simulink model "InteractiveArmModel_R2021a_v1"  (R2021a)
settings: Solver=ode4  StartTime=0.0  StopTime=3000  FixedStep=1/150  MaxStep=1/50  MinStep=1/200  RelTol=1e-5  AbsTol=1e-6  EnableMultiTasking=on
model workspace (MAT data in the model file):
  MaxEccentricFlexor = 0.5
  PoleZ = 0.85
  SampleTime = 0.05
  musNoise = 0
  musNoiseLevel : Simulink.Parameter (value not decoded)
libraries: simulink x1
(part 2 of 3)

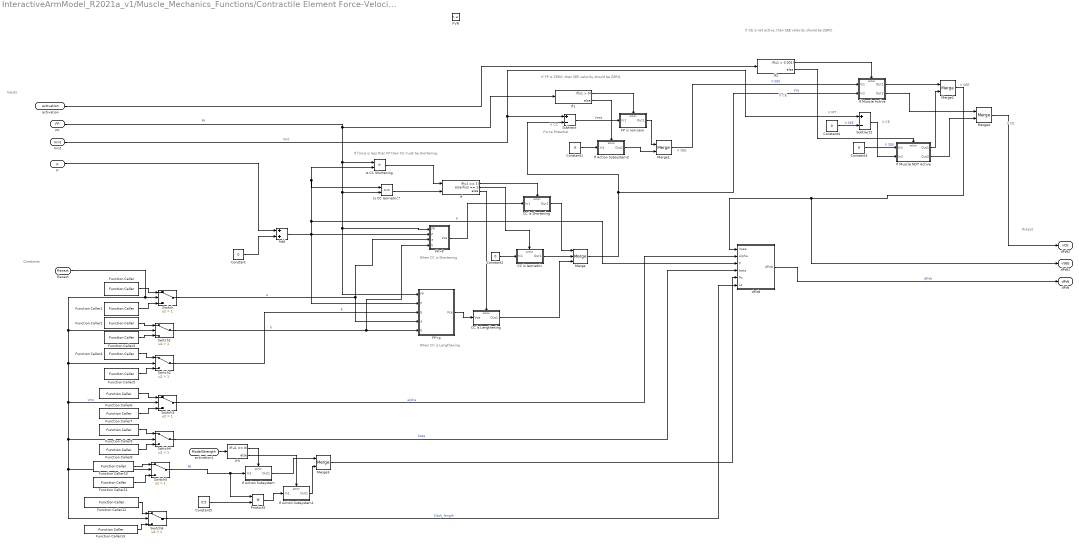
== system InteractiveArmModel_R2021a_v1/Muscle_Mechanics_Functions/Contractile Element Force-Velocity Relation ==
  note: V CE
  note: V MT
  note: V SEE
  note: V CE
  note: V CE
  note: V CC
  note: V SEE
  note: If force is less than FP then CC must be shortening.
  note: When CC is Shortening
  note: When CC is Lengthening
  note: Force Potential
  note: Output
  note: Inputs
  note: Constants
  note: If FP is ZERO, then SEE velocity should be ZERO.
  note: If CE is not active, then SEE velocity should be ZERO.
  FVR : TriggerPort  TriggerType=function-call  IsSimulinkFunction=on  FunctionName=FVR  FunctionVisibility=scoped  VariantControl=(inherit)
  Add : Sum
  CC is Isometric : Subsystem  TreatAsAtomicUnit=on
  CC is Lengthening : Subsystem  TreatAsAtomicUnit=on
  CC is Shortening : Subsystem  TreatAsAtomicUnit=on
  Constant{,1..4} (5 alike) : Constant  Value=0
  Constant5 : Constant  Value=0.5
  FP is non-zero : Subsystem  TreatAsAtomicUnit=on
  FP<p : Subsystem
  FP>P : Subsystem
  Function Caller : FunctionCaller  FunctionPrototype=y = Constants.aF()  InputArgumentSpecifications=<Enter example>  OutputArgumentSpecifications=<Enter example>
  Function Caller1 : FunctionCaller  FunctionPrototype=y = Constants.aE()  InputArgumentSpecifications=<Enter example>  OutputArgumentSpecifications=<Enter example>
  Function Caller10 : FunctionCaller  FunctionPrototype=y = Constants.P0F()  InputArgumentSpecifications=<Enter example>  OutputArgumentSpecifications=<Enter example>
  Function Caller11 : FunctionCaller  FunctionPrototype=y = Constants.P0E()  InputArgumentSpecifications=<Enter example>  OutputArgumentSpecifications=<Enter example>
  Function Caller12 : FunctionCaller  FunctionPrototype=y = Constants.Slack_lengthF()  InputArgumentSpecifications=<Enter example>  OutputArgumentSpecifications=<Enter example>
  Function Caller13 : FunctionCaller  FunctionPrototype=y = Constants.Slack_lengthE()  InputArgumentSpecifications=<Enter example>  OutputArgumentSpecifications=<Enter example>
  Function Caller2 : FunctionCaller  FunctionPrototype=y = Constants.bF()  InputArgumentSpecifications=<Enter example>  OutputArgumentSpecifications=<Enter example>
  Function Caller3 : FunctionCaller  FunctionPrototype=y = Constants.bE()  InputArgumentSpecifications=<Enter example>  OutputArgumentSpecifications=<Enter example>
  Function Caller4 : FunctionCaller  FunctionPrototype=y = Constants.EF()  InputArgumentSpecifications=<Enter example>  OutputArgumentSpecifications=<Enter example>
  Function Caller5 : FunctionCaller  FunctionPrototype=y = Constants.EE()  InputArgumentSpecifications=<Enter example>  OutputArgumentSpecifications=<Enter example>
  Function Caller6 : FunctionCaller  FunctionPrototype=y = Constants.alphaF()  InputArgumentSpecifications=<Enter example>  OutputArgumentSpecifications=<Enter example>
  Function Caller7 : FunctionCaller  FunctionPrototype=y = Constants.alphaE()  InputArgumentSpecifications=<Enter example>  OutputArgumentSpecifications=<Enter example>
  Function Caller8 : FunctionCaller  FunctionPrototype=y = Constants.betaE()  InputArgumentSpecifications=<Enter example>  OutputArgumentSpecifications=<Enter example>
  Function Caller9 : FunctionCaller  FunctionPrototype=y = Constants.betaF()  InputArgumentSpecifications=<Enter example>  OutputArgumentSpecifications=<Enter example>
  If : If  NumInputs=2  IfExpression=u1 == 1  ElseIfExpressions=u2 == 1
  If Action Subsystem : Subsystem  TreatAsAtomicUnit=on
  If Action Subsystem1 : Subsystem  TreatAsAtomicUnit=on
  If Action Subsystem3 : Subsystem  TreatAsAtomicUnit=on
  If Muscle Active : Subsystem  TreatAsAtomicUnit=on
  If Muscle NOT Active : Subsystem  TreatAsAtomicUnit=on
  If1 : If
  If2 : If  IfExpression=u1 > 0.001
  If3 : If  IfExpression=u1 == 0
  Is CC Isometric? : RelationalOperator  Operator===  OutDataTypeStr=boolean  RndMeth=Simplest
  Is CC Shortening : RelationalOperator  Operator=>  OutDataTypeStr=boolean  RndMeth=Simplest
  Merge : Merge  Inputs=3
  Merge{1..4} (4 alike) : Merge
  Product5 : Product
  Subtract : Sum  Inputs=+-
  Subtract2 : Sum  Inputs=+-
  Switch{,1..6} (7 alike) : Switch  Criteria=u2 > Threshold  Threshold=1
  dP/dt : Subsystem
  FP : ArgIn  DisableCoverage=on  ArgumentName=FP
  Vmt : ArgIn  DisableCoverage=on  Port=2  ArgumentName=Vmt
  p : ArgIn  DisableCoverage=on  Port=3  ArgumentName=p
  flexext : ArgIn  DisableCoverage=on  Port=4  ArgumentName=flexext
  activation : ArgIn  DisableCoverage=on  Port=5  ArgumentName=activation
  activation1 : ArgIn  DisableCoverage=on  Port=6  ArgumentName=ModelStrength
  dPdt1 : ArgOut  DisableCoverage=on  ArgumentName=vSEE
  dPdt : ArgOut  DisableCoverage=on  Port=2  ArgumentName=dPdt
  dPdt2 : ArgOut  DisableCoverage=on  Port=3  ArgumentName=vCE
  wires:
  FP/1 -> If1/1, Is CC Shortening/1, Is CC Isometric?/2, FP<p/1(FP), FP>P/1(FP)  "FP"
  Switch2/1 -> FP<p/3(E)  "E"
  Switch1/1 -> FP>P/4(b), FP<p/5(b)  "b"
  FP<p/1(Vce) -> CC is Lengthening/1(Vce)
  FP>P/1(Vce) -> CC is Shortening/1(In1)
  Merge/1 -> If Muscle Active/2(In2), Subtract/2  "Vce"
  Switch/1 -> FP>P/3(a), FP<p/4(a)  "a"
  If/1 -> CC is Shortening/Action
  dP/dt/1(dP/dt) -> dPdt/1  "dP/dt"
  Switch4/1 -> dP/dt/4(beta)  "beta"
  If/3 -> CC is Lengthening/Action
  Is CC Shortening/1 -> If/1
  Switch3/1 -> dP/dt/2(alpha)  "alpha"
  Constant/1 -> Add/2
  CC is Shortening/1(Out1) -> Merge/1
  Switch6/1 -> dP/dt/6(Ls)  "Slack_length"
  Vmt/1 -> Subtract2/1, Subtract/1  "Vmt"
  CC is Lengthening/1(Out1) -> Merge/3
  Is CC Isometric?/1 -> If/2
  If/2 -> CC is Isometric/Action
  Constant2/1 -> CC is Isometric/1(In1)
  p/1 -> Add/1
  Function Caller1/1 -> Switch/3
  Function Caller/1 -> Switch/1
  flexext/1 -> Switch/2, Switch5/2, Switch6/2, Switch4/2, Switch3/2, Switch2/2, Switch1/2  "Vmt"
  Function Caller2/1 -> Switch1/1
  Function Caller3/1 -> Switch1/3
  Function Caller4/1 -> Switch2/1
  Function Caller5/1 -> Switch2/3
  Function Caller6/1 -> Switch3/1
  Function Caller7/1 -> Switch3/3
  Function Caller9/1 -> Switch4/1
  Function Caller8/1 -> Switch4/3
  Function Caller10/1 -> Switch5/1
  Function Caller11/1 -> Switch5/3
  Function Caller13/1 -> Switch6/3
  Function Caller12/1 -> Switch6/1
  Subtract/1 -> FP is non-zero/1(In1)  "Vsee"
  If1/1 -> FP is non-zero/Action
  If1/2 -> If Action Subsystem3/Action
  Constant1/1 -> If Action Subsystem3/1(In1)
  FP is non-zero/1(Out1) -> Merge1/1
  If Action Subsystem3/1(Out1) -> Merge1/2
  activation/1 -> If2/1
  If2/1 -> If Muscle Active/Action
  If2/2 -> If Muscle NOT Active/Action
  Merge1/1 -> If Muscle Active/1(In1)  "V SEE"
  Constant3/1 -> If Muscle NOT Active/1(In1)  "V SEE"
  If Muscle Active/1(Out1) -> Merge2/1
  If Muscle NOT Active/1(Out1) -> Merge2/2
  Merge2/1 -> dPdt1/1, dP/dt/1(Vsee)
  CC is Isometric/1(Out1) -> Merge/2
  Add/1 -> Is CC Shortening/2, Is CC Isometric?/1, dP/dt/3(P), FP<p/2(P), FP>P/2(P)  "P"
  Subtract2/1 -> If Muscle NOT Active/2(In2)
  If Muscle Active/2(Out2) -> Merge4/1
  If Muscle NOT Active/2(Out2) -> Merge4/2
  Merge4/1 -> dPdt2/1
  Constant4/1 -> Subtract2/2  "V SEE"
  Merge3/1 -> dP/dt/5(Po)
  Switch5/1 -> Product5/1, If Action Subsystem/1(In1)  "P0"
  activation1/1 -> If3/1
  If3/1 -> If Action Subsystem/Action
  If Action Subsystem/1(Out1) -> Merge3/1
  Constant5/1 -> Product5/2
  Product5/1 -> If Action Subsystem1/1(In1)
  If3/2 -> If Action Subsystem1/Action
  If Action Subsystem1/1(Out1) -> Merge3/2

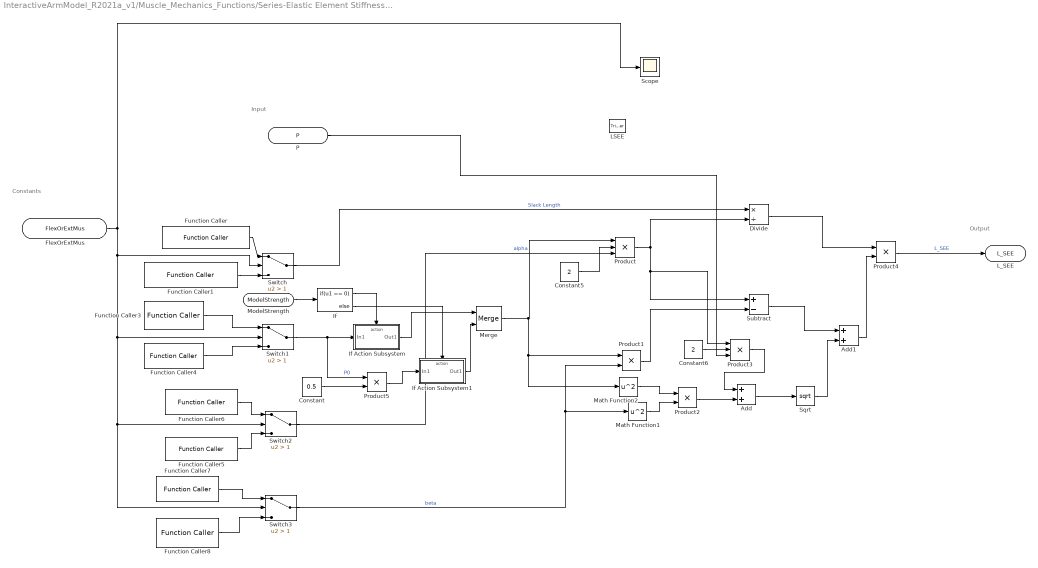
== system InteractiveArmModel_R2021a_v1/Muscle_Mechanics_Functions/Series-Elastic Element Stiffness Relation  ==
  note: Output
  note: Input
  note: Constants
  LSEE : TriggerPort  TriggerType=function-call  IsSimulinkFunction=on  FunctionName=LSEE  FunctionVisibility=scoped  VariantControl=(inherit)
  Add : Sum
  Add1 : Sum
  Constant : Constant  Value=0.5
  Constant5 : Constant  Value=2
  Constant6 : Constant  Value=2
  Divide : Product  Inputs=*/
  Function Caller : FunctionCaller  FunctionPrototype=y = Constants.Slack_lengthF()  InputArgumentSpecifications=<Enter example>  OutputArgumentSpecifications=<Enter example>
  Function Caller1 : FunctionCaller  FunctionPrototype=y = Constants.Slack_lengthE()  InputArgumentSpecifications=<Enter example>  OutputArgumentSpecifications=<Enter example>
  Function Caller3 : FunctionCaller  FunctionPrototype=y = Constants.P0F()  InputArgumentSpecifications=<Enter example>  OutputArgumentSpecifications=<Enter example>
  Function Caller4 : FunctionCaller  FunctionPrototype=y = Constants.P0E()  InputArgumentSpecifications=<Enter example>  OutputArgumentSpecifications=<Enter example>
  Function Caller5 : FunctionCaller  FunctionPrototype=y = Constants.alphaE()  InputArgumentSpecifications=<Enter example>  OutputArgumentSpecifications=<Enter example>
  Function Caller6 : FunctionCaller  FunctionPrototype=y = Constants.alphaF()  InputArgumentSpecifications=<Enter example>  OutputArgumentSpecifications=<Enter example>
  Function Caller7 : FunctionCaller  FunctionPrototype=y = Constants.betaF()  InputArgumentSpecifications=<Enter example>  OutputArgumentSpecifications=<Enter example>
  Function Caller8 : FunctionCaller  FunctionPrototype=y = Constants.betaE()  InputArgumentSpecifications=<Enter example>  OutputArgumentSpecifications=<Enter example>
  If : If  IfExpression=u1 == 0
  If Action Subsystem : Subsystem  TreatAsAtomicUnit=on
  If Action Subsystem1 : Subsystem  TreatAsAtomicUnit=on
  Math Function1 : Math  Operator=square  SaturateOnIntegerOverflow=on
  Math Function2 : Math  Operator=square  SaturateOnIntegerOverflow=on
  Merge : Merge
  Product : Product  Inputs=3
  Product{1..2,4..5} (4 alike) : Product
  Product3 : Product  Inputs=3
  Scope : Scope
  Sqrt : Sqrt  SaturateOnIntegerOverflow=on
  Subtract : Sum  Inputs=+-
  Switch{,1..3} (4 alike) : Switch  Criteria=u2 > Threshold  Threshold=1
  P : ArgIn  DisableCoverage=on  ArgumentName=P
  FlexOrExtMus : ArgIn  DisableCoverage=on  Port=2  ArgumentName=FlexOrExtMus
  ModelStrength : ArgIn  DisableCoverage=on  Port=3  ArgumentName=ModelStrength
  L_SEE : ArgOut  DisableCoverage=on  ArgumentName=L_SEE
  wires:
  P/1 -> Product3/3
  Product3/1 -> Add/1
  Product2/1 -> Add/2
  Math Function2/1 -> Product2/1
  Constant5/1 -> Product/2
  Product4/1 -> L_SEE/1  "L_SEE"
  Constant6/1 -> Product3/2
  Product/1 -> Divide/2, Product3/1, Subtract/1
  Sqrt/1 -> Add1/2
  Add1/1 -> Product4/2
  Switch3/1 -> Math Function1/1, Product1/2  "beta"
  Subtract/1 -> Add1/1
  Switch2/1 -> Product/3  "alpha"
  Math Function1/1 -> Product2/2
  Add/1 -> Sqrt/1
  Switch/1 -> Divide/1  "Slack Length"
  Divide/1 -> Product4/1
  Product1/1 -> Subtract/2
  Function Caller/1 -> Switch/1
  Function Caller1/1 -> Switch/3
  Function Caller3/1 -> Switch1/1
  Function Caller4/1 -> Switch1/3
  Function Caller6/1 -> Switch2/1
  Function Caller5/1 -> Switch2/3
  Function Caller8/1 -> Switch3/3
  Function Caller7/1 -> Switch3/1
  FlexOrExtMus/1 -> Switch3/2, Switch2/2, Switch1/2, Switch/2, Scope/1
  ModelStrength/1 -> If/1
  Switch1/1 -> Product5/1, If Action Subsystem/1(In1)  "P0"
  If/1 -> If Action Subsystem/Action
  If/2 -> If Action Subsystem1/Action
  Constant/1 -> Product5/2
  Product5/1 -> If Action Subsystem1/1(In1)
  If Action Subsystem/1(Out1) -> Merge/1
  If Action Subsystem1/1(Out1) -> Merge/2
  Merge/1 -> Math Function2/1, Product1/1, Product/1

== system InteractiveArmModel_R2021a_v1/Trial Start//Stop//Increment Control/Counter for Trial Number ==
  Trigger : TriggerPort  VariantControl=Variant
  Add : Sum
  Constant : Constant  Value=0
  Delay : Delay  DelayLength=1  InitialCondition=0
  Increment Stored Integer : simulink/Additional Math & Discrete/Additional Math: Increment - Decrement/Increment Stored Integer
  Trial Number Switch : Outport
  wires:
  Constant/1 -> Add/1
  Add/1 -> Increment Stored Integer/1
  Increment Stored Integer/1 -> Trial Number Switch/1, Delay/1
  Delay/1 -> Add/2

== system InteractiveArmModel_R2021a_v1/Trial Start//Stop//Increment Control/Extract Movement Time ==
  Trial Time : Inport
  Loop Running Flag : TriggerPort  TriggerType=falling  VariantControl=Variant
  Movement Time : Outport
  wires:
  Trial Time/1 -> Movement Time/1

== system InteractiveArmModel_R2021a_v1/Trial Start//Stop//Increment Control/Flag for What Phase Trial is In ==
  note: Flags
      | Specifying
      | What
      | Phase of Trial
      | Is Model
      | Currentely In
  Trial Time Flag : Inport
  Stop Criteria Flag : Inport  Port=2
  If Action Subsystem5 : Subsystem  TreatAsAtomicUnit=on
  If Action Subsystem6 : Subsystem  TreatAsAtomicUnit=on
  If Action Subsystem7 : Subsystem  TreatAsAtomicUnit=on
  If3 : If  NumInputs=2  IfExpression=u1 == 0  ElseIfExpressions=u2 == 0
  Merge2 : Merge  Inputs=3
  StopCriteriaFlag : Constant  Value=2
  TrialIsRunning : Constant  Value=0
  TrialTimeFlag : Constant
  message display : Outport
  wires:
  If Action Subsystem6/1(Out1) -> Merge2/2
  If Action Subsystem7/1(Out1) -> Merge2/3
  If Action Subsystem5/1(Out1) -> Merge2/1
  TrialTimeFlag/1 -> If Action Subsystem5/1(In1)  "Time is up"
  TrialIsRunning/1 -> If Action Subsystem7/1(In1)  "Keeps running"
  Stop Criteria Flag/1 -> If3/2
  If3/2 -> If Action Subsystem6/Action
  If3/1 -> If Action Subsystem5/Action
  StopCriteriaFlag/1 -> If Action Subsystem6/1(In1)  "Success"
  If3/3 -> If Action Subsystem7/Action
  Trial Time Flag/1 -> If3/1
  Merge2/1 -> message display/1  "message display"

== system InteractiveArmModel_R2021a_v1/Trial Start//Stop//Increment Control/Reset Trigger Logic ==
  note: Reset Trigger
  Trial Time : Inport
  Stop Criteria Flag : Inport  Port=2
  Constant1 : Constant  Value=0
  Logical Operator1 : Logic  AllPortsSameDT=off  OutDataTypeStr=boolean
  Relational Operator : RelationalOperator  Operator=>  OutDataTypeStr=boolean  RndMeth=Simplest
  Reset Trigger : Outport
  wires:
  Relational Operator/1 -> Logical Operator1/1
  Trial Time/1 -> Relational Operator/1
  Constant1/1 -> Relational Operator/2
  Stop Criteria Flag/1 -> Logical Operator1/2
  Logical Operator1/1 -> Reset Trigger/1  "Reset Trigger"

== system InteractiveArmModel_R2021a_v1/Trial Start//Stop//Increment Control/Stop Criteria Flag Control (Between Trials) ==
  note: Immediately goes to zero when stop on target. Switches to 1 at the start of the one-second "get ready" pre-trial wait time.
  note: 0 = Stop criteria Satisfied.
  note: Detect 0 at Stop Criteria, wait for a second, and make that 1 again. If the trial (while loop)
      |  is stopped because of the StopCriteria, this logic makes it start again for the next trial
  Stop Criteria Flag In : Inport
  Constant : Constant
  Data Type Conversion1 : DataTypeConversion
  Delay1 : Delay  DelayLength=100  InitialCondition=0
  Delay2 : Delay  DelayLength=1  InitialCondition=0
  If Action Subsystem3 : Subsystem  TreatAsAtomicUnit=on
  If Action Subsystem4 : Subsystem  TreatAsAtomicUnit=on
  If2 : If  IfExpression=u1 == 0
  Merge1 : Merge
  Stop Criteria Flag Out : Outport
  wires:
  Stop Criteria Flag In/1 -> Delay2/1, Delay1/1
  If Action Subsystem3/1(Out1) -> Merge1/1
  If Action Subsystem4/1(Out1) -> Merge1/2
  If2/1 -> If Action Subsystem3/Action
  Delay1/1 -> If2/1
  Merge1/1 -> Stop Criteria Flag Out/1  "StopCriteria"
  Data Type Conversion1/1 -> If Action Subsystem4/1(In1)
  Delay2/1 -> Data Type Conversion1/1
  If2/2 -> If Action Subsystem4/Action
  Constant/1 -> If Action Subsystem3/1(In1)

== system InteractiveArmModel_R2021a_v1/Trial Start//Stop//Increment Control/Subsystem ==
  note: If 0, then trial time is up or stop criteria is satisfied, so reset the trial time to 0.
  note: Reset the trial time for each trial.
  In1 : Inport
  Digital Clock : DigitalClock  SampleTime=-1
  If : If  IfExpression=u1 == 0  ShowElse=off
  If Action Subsystem : Subsystem  TreatAsAtomicUnit=on
  Subtract : Sum  Inputs=+-
  To Workspace1 : ToWorkspace  VariableName=simulationTime  SampleTime=-1
  To Workspace2 : ToWorkspace  VariableName=trialTime  SampleTime=-1
  Simulation Time : Outport
  Trial Time : Outport  Port=2
  wires:
  Digital Clock/1 -> Simulation Time/1, Subtract/1, If Action Subsystem/1(In1), To Workspace1/1
  If Action Subsystem/1(Out1) -> Subtract/2
  Subtract/1 -> Trial Time/1, To Workspace2/1  "Trial time"
  If/1 -> If Action Subsystem/Action
  In1/1 -> If/1

== system InteractiveArmModel_R2021a_v1/Trial Start//Stop//Increment Control/Subsystem1 ==
  note: Changes to zero if trial time exceeded.
  note: StopCriteria&TrialTime
  Trial Time : Inport
  Stop Criteria Flag : Inport  Port=2
  Logical Operator : Logic  AllPortsSameDT=off  OutDataTypeStr=boolean
  Product : Product
  Relational Operator2 : RelationalOperator  Operator=<  RndMeth=Simplest
  Trial time : Constant  Value=5
  Trial time1 : Constant
  StopCriteria&TrialTime Flag : Outport
  Trial Time Flag : Outport  Port=2
  wires:
  Trial time1/1 -> Product/1
  Relational Operator2/1 -> Product/2
  Stop Criteria Flag/1 -> Logical Operator/2
  Logical Operator/1 -> StopCriteria&TrialTime Flag/1  "StopCriteria&TrialTime"
  Trial time/1 -> Relational Operator2/2
  Product/1 -> Trial Time Flag/1, Logical Operator/1  "Time"
  Trial Time/1 -> Relational Operator2/1

== system InteractiveArmModel_R2021a_v1/Trial Start//Stop//Increment Control/Subsystem2 ==
  note: Make IC 1 for the first 0.01 sec. This is to start the trials.
  Simulation Time : Inport
  StopCriteria&TrialTime Flag : Inport  Port=2
  Constant2 : Constant
  If Action Subsystem1 : Subsystem  TreatAsAtomicUnit=on
  If Action Subsystem2 : Subsystem  TreatAsAtomicUnit=on
  If1 : If  IfExpression=u1 < 0.01
  Merge : Merge
  Product1 : Product
  Trial time2 : Constant
  IC : Outport
  wires:
  If1/1 -> If Action Subsystem1/Action
  Constant2/1 -> If Action Subsystem1/1(In1)
  StopCriteria&TrialTime Flag/1 -> Product1/1
  If Action Subsystem1/1(Out1) -> Merge/1
  If Action Subsystem2/1(Out1) -> Merge/2
  Trial time2/1 -> Product1/2
  Merge/1 -> IC/1  "IC"
  Product1/1 -> If Action Subsystem2/1(In1)  "Time"
  If1/2 -> If Action Subsystem2/Action
  Simulation Time/1 -> If1/1

== system InteractiveArmModel_R2021a_v1/While Loop (Main Simulation Code)/Actuator Selection Logic ==
  Control Input : Inport
  Add2 : Sum
  Constant{,1..3,5..6} (6 alike) : Constant  Value=0
  Constant4 : Constant
  Function Caller : FunctionCaller  FunctionPrototype=y = Constants.ActuatorType()  InputArgumentSpecifications=<Enter example>  OutputArgumentSpecifications=<Enter example>
  Multiport Switch : MultiPortSwitch
  Multiport Switch1 : MultiPortSwitch
  Multiport Switch2 : MultiPortSwitch
  Torque Control Signal : Outport
  Force Actuator Control Signal : Outport  Port=2
  MuscleControlSignal : Outport  Port=3
  wires:
  Add2/1 -> Multiport Switch/1, Multiport Switch2/1, Multiport Switch1/1
  Constant2/1 -> Multiport Switch1/2
  Control Input/1 -> Multiport Switch/4, Multiport Switch1/3, Multiport Switch2/2
  Constant6/1 -> Multiport Switch2/4
  Constant4/1 -> Add2/2
  Constant1/1 -> Multiport Switch/3
  Function Caller/1 -> Add2/1
  Constant/1 -> Multiport Switch/2
  Constant5/1 -> Multiport Switch1/4
  Constant3/1 -> Multiport Switch2/3
  Multiport Switch1/1 -> Force Actuator Control Signal/1
  Multiport Switch/1 -> Torque Control Signal/1
  Multiport Switch2/1 -> MuscleControlSignal/1

== system InteractiveArmModel_R2021a_v1/While Loop (Main Simulation Code)/Force Gen. ==
  Force(F&E) : Inport
  Demux : Demux  Outputs=2
  Ext Actuator Strength : Constant  Value=10
  Flex Actuator Strength : Constant  Value=10
  Mux : Mux  Inputs=2
  Product : Product
  Product1 : Product
  Extensor Force : Outport
  wires:
  Demux/2 -> Product/1  "Extensor force (N)"
  Product/1 -> Mux/2  "Extensor force"
  Ext Actuator Strength/1 -> Product/2
  Demux/1 -> Product1/1  "Flexor force (N)"
  Flex Actuator Strength/1 -> Product1/2
  Product1/1 -> Mux/1  "Flexor force"
  Force(F&E)/1 -> Demux/1
  Mux/1 -> Extensor Force/1

== system InteractiveArmModel_R2021a_v1/While Loop (Main Simulation Code)/Force//Torque Conversion ==
  note: If Selector = 2 Then Torque Control
  note: Convert Force Gen. to Torque
  note: Force Generator Input
  note: Moment Arm Input
  note: Muscle Model Force Input
  note: Torque Input
  note: If Selector = 1 Then Force Control
  note: If Selector = 1 Then Force Control
  note: If Selector = 0 Then Muscle Control
  Torque : Inport
  Force 1 : Inport  Port=2
  Force 2 : Inport  Port=3
  MA : Inport  Port=4
  Add : Sum
  Demux{,1..3} (4 alike) : Demux  Outputs=2
  Display : Display
  Function Caller : FunctionCaller  FunctionPrototype=y = Constants.ActuatorType()  InputArgumentSpecifications=<Enter example>  OutputArgumentSpecifications=<Enter example>
  Generator PE : Switch  Criteria=u2 > Threshold
  Generator PF : Switch  Criteria=u2 > Threshold
  "Generator TE " : Switch  Criteria=u2 > Threshold  Threshold=1
  Generator TF : Switch  Criteria=u2 > Threshold  Threshold=1
  Product7 : Product
  Product8 : Product
  To Workspace1 : ToWorkspace  VariableName=actuatorTorqueExt  SaveFormat=Timeseries  SampleTime=-1
  To Workspace3 : ToWorkspace  VariableName=actuatorTorqueFlex  SaveFormat=Timeseries  SampleTime=-1
  Mus Torque : Outport
  wires:
  "Generator TE "/1 -> To Workspace1/1, Add/2  "Extensor Torque"
  Demux1/1 -> Generator PF/1  "Flexor Force"
  Demux3/1 -> Generator PF/3, Display/1  "P Flexor"
  Add/1 -> Mus Torque/1  "Net Muscular torque"
  Demux1/2 -> Generator PE/1  "Extensor Force"
  Generator PE/1 -> Product8/1  "Extensor Force"
  Demux3/2 -> Generator PE/3  "P Extensor"
  Generator TF/1 -> To Workspace3/1, Add/1  "Flexor Torque"
  Demux2/1 -> Generator TF/1  "Flexor Torque"
  Demux2/2 -> "Generator TE "/1  "Extensor Torque"
  Demux/1 -> Product8/2  "Extensor Moment Arm"
  MA/1 -> Demux/1
  Force 1/1 -> Demux1/1
  Torque/1 -> Demux2/1
  Force 2/1 -> Demux3/1
  Product7/1 -> Generator TF/3  "Flexor Torque"
  Demux/2 -> Product7/2  "Flexor Moment Arm"
  Generator PF/1 -> Product7/1
  Product8/1 -> "Generator TE "/3  "Extansor Torque"
  Function Caller/1 -> Generator PE/2, "Generator TE "/2, Generator TF/2, Generator PF/2

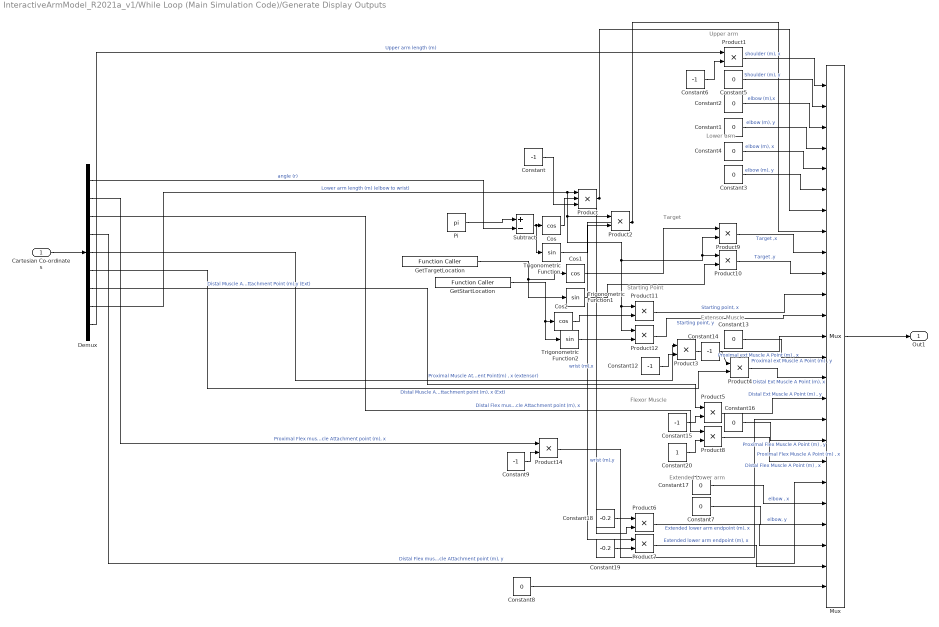
== system InteractiveArmModel_R2021a_v1/While Loop (Main Simulation Code)/Generate Display Outputs ==
  note: Extended Lower arm
  note: Flexor Muscle
  note: Extensor Muscle
  note: Starting
      | Point
  note: Target
  note: Lower
      | arm
  note: Upper arm
  Cartesian Co-ordinates : Inport
  Constant{,6,9,12,14..15} (6 alike) : Constant  Value=-1
  Constant{1..5,7..8,13,16..17} (10 alike) : Constant  Value=0
  Constant18 : Constant  Value=-0.2
  Constant19 : Constant  Value=-0.2
  Constant20 : Constant
  Cos : Trigonometry  Operator=cos
  Cos1 : Trigonometry  Operator=cos
  Cos2 : Trigonometry  Operator=cos
  Demux : Demux  Outputs=9
  GetStartLocation : FunctionCaller  FunctionPrototype=y = Constants.startLoc()  InputArgumentSpecifications=<Enter example>  OutputArgumentSpecifications=<Enter example>
  GetTargetLocation : FunctionCaller  FunctionPrototype=y = Constants.targetLoc()  InputArgumentSpecifications=<Enter example>  OutputArgumentSpecifications=<Enter example>
  Mux : Mux  Inputs=25
  Pi : Constant  Value=pi  OutDataTypeStr=Inherit: Inherit via back propagation
  Product : Product  Inputs=3
  Product{1..12,14} (13 alike) : Product
  Subtract : Sum  Inputs=+-
  Trigonometric Function : Trigonometry
  Trigonometric Function1 : Trigonometry
  Trigonometric Function2 : Trigonometry
  Out1 : Outport
  wires:
  Constant13/1 -> Mux/14  "Proximal ext Muscle A Point (m) , y"
  Constant12/1 -> Product3/2
  Product10/1 -> Mux/10  "Target ,y"
  Constant15/1 -> Product5/2
  Constant5/1 -> Mux/2  "Shoulder (m), y"
  Product4/1 -> Mux/15  "Distal Ext Muscle A Point (m), x"
  Product9/1 -> Mux/9  "Target ,x"
  Constant6/1 -> Product1/2
  Subtract/1 -> Trigonometric Function/1, Cos/1
  Demux/7 -> Product5/1  "Distal Muscle Attachment Point (m),y (Ext)"
  Product5/1 -> Mux/16  "Distal Ext Muscle A Point (m) , y"
  Product1/1 -> Mux/1  "shoulder (m), x"
  Product11/1 -> Mux/11  "Starting point, x"
  Product3/1 -> Mux/13  "Proximal ext Muscle A Point (m) , x"
  Product12/1 -> Mux/12  "Starting point, y"
  Constant14/1 -> Product4/1
  Demux/6 -> Product4/2  "Distal Muscle Attachment point (m), x (Ext)"
  Demux/5 -> Product3/1  "Proximal Muscle Attachment Point(m) , x (extensor)"
  Demux/9 -> Product1/1  "Upper arm length (m)"
  Constant16/1 -> Mux/18  "Proximal Flex Muscle A Point (m) , y"
  Pi/1 -> Subtract/1
  Demux/1 -> Subtract/2  "angle (r)"
  Constant1/1 -> Mux/4  "elbow (m), y"
  Constant2/1 -> Mux/3  "elbow (m),x"
  Cos/1 -> Product/2
  Product/1 -> Mux/7, Product6/2  "wrist (m),x"
  Trigonometric Function/1 -> Product2/2
  Product2/1 -> Mux/8, Product7/1  "wrist (m),y"
  Constant/1 -> Product/3
  Constant17/1 -> Mux/21  "elbow , x"
  Constant7/1 -> Mux/22  "elbow, y"
  Constant18/1 -> Product6/1
  Constant19/1 -> Product7/2
  Product6/1 -> Mux/23  "Extended lower arm endpoint (m), x"
  Product7/1 -> Mux/24  "Extended lower arm endpoint (m), x"
  Constant20/1 -> Product8/2
  Product8/1 -> Mux/19  "Distal Flex Muscle A Point (m) , x"
  Demux/8 -> Product/1, Product9/2, Product10/1, Product12/1, Product11/1, Product2/1  "Lower arm length (m) (elbow to wrist)"
  GetTargetLocation/1 -> Cos1/1, Trigonometric Function1/1
  Cos1/1 -> Product9/1
  Trigonometric Function1/1 -> Product10/2
  GetStartLocation/1 -> Trigonometric Function2/1, Cos2/1
  Cos2/1 -> Product11/2
  Trigonometric Function2/1 -> Product12/2
  Product14/1 -> Mux/17  "Proximal Flex Muscle A Point (m) , x"
  Constant4/1 -> Mux/5  "elbow (m), x"
  Constant3/1 -> Mux/6  "elbow (m), y"
  Demux/2 -> Product14/1  "Proximal Flex muscle Attachment point (m), x"
  Constant9/1 -> Product14/2
  Demux/3 -> Product8/1  "Distal Flex muscle Attachment point (m), x"
  Demux/4 -> Mux/20  "Distal Flex muscle Attachment point (m), y"
  Cartesian Co-ordinates/1 -> Demux/1
  Mux/1 -> Out1/1
  Constant8/1 -> Mux/25

== system InteractiveArmModel_R2021a_v1/While Loop (Main Simulation Code)/Integrator 1 ==
  Reset1 : Inport
  Arm Accel. : Inport  Port=2
  Integrater : Subsystem
  Reset : Subsystem
  Reset2 : Subsystem
  Arm Vel. : Outport
  wires:
  Reset/1(Accel) -> Integrater/1(Accel)
  Arm Accel./1 -> Reset/2(" Accel")
  Reset1/1 -> Reset2/1(Reset), Reset/1(Reset)
  Integrater/1(Vel) -> Reset2/2(VelIn)  "Arm Vel."
  Reset2/1(VelOut) -> Arm Vel./1  "Velocity"

== system InteractiveArmModel_R2021a_v1/While Loop (Main Simulation Code)/Integrator 2 ==
  Reset : Inport
  Arm Vel. : Inport  Port=2
  Integrater 1 : Subsystem
  Reset2 : Subsystem
  PosOut : Outport
  wires:
  Reset/1 -> Reset2/1(Reset)
  Arm Vel./1 -> Integrater 1/1(VelIn)  "Velocity"
  Integrater 1/1(PosOut) -> Reset2/2(PosIn)  "Position"
  Reset2/1(PosOut) -> PosOut/1

== system InteractiveArmModel_R2021a_v1/While Loop (Main Simulation Code)/Muscle Models ==
  Excitation(flex+Ext) : Inport
  IC : Inport  Port=2
  Lmt(flex+Ext) : Inport  Port=3
  Add Noise to Keyboard / Mouse Control Input Types : Subsystem
  BangBangConst1 : Constant  Value=0.1
  Demux : Demux  Outputs=2
  Demux1 : Demux  Outputs=2
  EMG Calibration1 : Subsystem
  EMG Control : Subsystem  TreatAsAtomicUnit=on
  Extensor Muscle Mechanics : Subsystem
  Flexor Muscle Mechanics : Subsystem
  Function Caller : FunctionCaller  FunctionPrototype=y = Constants.ModelStrengthControl()  InputArgumentSpecifications=<Enter example>  OutputArgumentSpecifications=<Enter example>
  If1 : If  IfExpression=u1 == 0  ElseIfExpressions=u1 == 1, u1 == 2  ShowElse=off
  Keyboard / Mouse / EMG Control Mode : FunctionCaller  FunctionPrototype=y = Constants.ControlMode()  OutputArgumentSpecifications=<Enter example>
  Keyboard Control : Subsystem  TreatAsAtomicUnit=on
  Merge1 : Merge  Inputs=3
  Mouse Control : Subsystem  TreatAsAtomicUnit=on
  Mux : Mux  Inputs=2
  Product1 : Product
  Product2 : Product
  To Workspace : ToWorkspace  VariableName=calibratedMusStimFlex  SaveFormat=Timeseries  SampleTime=-1
  To Workspace11 : ToWorkspace  VariableName=calibratedMusStimExt  SaveFormat=Timeseries  SampleTime=-1
  To Workspace12 : ToWorkspace  VariableName=muscleForce  SaveFormat=Timeseries  SampleTime=-1
  Muscle Force (Ext+Flex) : Outport
  wires:
  If1/3 -> EMG Control/Action
  Excitation(flex+Ext)/1 -> EMG Calibration1/1(stimulation(flex+Ext)), Add Noise to Keyboard / Mouse Control Input Types/1(In1)
  Function Caller/1 -> Flexor Muscle Mechanics/4(ModelAge), Extensor Muscle Mechanics/4(ModelAge)
  Mouse Control/1(Out1) -> Merge1/2
  Demux1/2 -> To Workspace11/1, Extensor Muscle Mechanics/1("Excitation Extensor ")  "Excitation Extensor"
  Merge1/1 -> Demux1/1  "Excitation"
  Add Noise to Keyboard / Mouse Control Input Types/1(Out1) -> Product2/2, Product1/1
  BangBangConst1/1 -> Product2/1, Product1/2
  EMG Calibration1/1(Excitation (Range: 0-1)) -> EMG Control/1(stimulation(flex+Ext))
  Product2/1 -> Mouse Control/1(stimulation(flex+Ext))
  Extensor Muscle Mechanics/1(P Extenasor) -> Mux/2  "Extenasor Force (N)"
  Product1/1 -> Keyboard Control/1(stimulation(flex+Ext))
  EMG Control/1(Out1) -> Merge1/3
  Demux1/1 -> To Workspace/1, Flexor Muscle Mechanics/1(ExcitationFlexor)  "Excitation Flexor"
  IC/1 -> Flexor Muscle Mechanics/2(IC), Extensor Muscle Mechanics/2(IC)
  If1/2 -> Mouse Control/Action
  If1/1 -> Keyboard Control/Action
  Lmt(flex+Ext)/1 -> Demux/1
  Keyboard Control/1(Out1) -> Merge1/1
  Demux/2 -> Flexor Muscle Mechanics/3(LmtFlexor)  "LMT Flexor"
  Keyboard / Mouse / EMG Control Mode/1 -> If1/1
  Demux/1 -> Extensor Muscle Mechanics/3(LMT Extensor)  "LMT Extensor"
  Flexor Muscle Mechanics/1(P Flexor) -> Mux/1  "Flexor Force (N)"
  Mux/1 -> To Workspace12/1, Muscle Force (Ext+Flex)/1

== system InteractiveArmModel_R2021a_v1/While Loop (Main Simulation Code)/Musculoskeletal Geometry ==
  angle (radians) : Inport
  LMT Extensor : Subsystem
  LMT Flexor : Subsystem
  "Lower arm length (m) " : Constant  Value=0.3
  MA Extensor : Subsystem
  MA Flexor : Subsystem
  Mux : Mux  Inputs=9
  Mux1 : Mux  Inputs=2
  Mux2 : Mux  Inputs=2
  Upper Arm length (m) : Constant  Value=0.38
  MA (Flex+Ext) : Outport
  Cartesian Co-ordinates : Outport  Port=2
  Lmt (Flex+Ext) : Outport  Port=3
  wires:
  Upper Arm length (m)/1 -> Mux/9, LMT Flexor/3(upper arm length (m)), MA Extensor/4(Upper arm length (m)), MA Flexor/4(Upper arm length (m)), LMT Extensor/3(upper arm length (m))  "Upper arm length (m)"
  angle (radians)/1 -> Mux/1, MA Flexor/1(angle (radians)), MA Extensor/1(angle (radians)), LMT Extensor/1(angle (r)), LMT Flexor/1(angle (r))  "angle (radians)1"
  LMT Flexor/1(Lmt Flexor (m)) -> Mux1/2, MA Flexor/2(Lmt Extensor (m))  "Flexor LMT (m)"
  "Lower arm length (m) "/1 -> Mux/8, LMT Extensor/2(Lower Arm length (m)), MA Extensor/3(lower arm length (m)), MA Flexor/3(Lower arm length (m)), LMT Flexor/2(lower arm length (m))  "Lower arm Length (m)"
  MA Flexor/1(Flexor moment arm (m)) -> Mux2/2  "Flexor  MA (m)"
  MA Extensor/1(Extensor Moment arm (m)) -> Mux2/1  "Extensor MA (m)"
  LMT Flexor/3("Distal Flex muscle Attachment (m), x") -> Mux/3  "Distal Flexor Muscle Attachment point (m), x"
  LMT Extensor/1(Lmt Extensor (m)) -> Mux1/1, MA Extensor/2(Lmt Extensor (m))  "Extensor LMT (m)"
  LMT Extensor/2(Proximal Ext Muscle attachment (m),x) -> Mux/5  "Proximal Muscle Attachment Point (m), x (fExtensor))"
  LMT Extensor/4(Distal Ext Muscle Attachment (m) ,y) -> Mux/7  "Distal Muscle Attachment Point (m) ,y (Ext)"
  LMT Extensor/3(Distal Ext Muscle Attachment (m) ,x) -> Mux/6  "Distal Muscle Attachment point (m), x (Ext)"
  LMT Flexor/2("Proximal Flex muscle Attachment (m), x ") -> Mux/2  "Proximal Flexor Muscle attachment point (m), x"
  LMT Flexor/4("Distal Flex muscle Attachment (m), y ") -> Mux/4  "Distal Flex0r muscle Attachment point (m), y"
  Mux/1 -> Cartesian Co-ordinates/1
  Mux1/1 -> Lmt (Flex+Ext)/1
  Mux2/1 -> MA (Flex+Ext)/1

== system InteractiveArmModel_R2021a_v1/While Loop (Main Simulation Code)/Passive External Torques ==
  Position : Inport
  Velocity : Inport  Port=2
  Add : Sum
  Global Damping : Constant  Value=-0.3
  Passive torque : Subsystem
  Product3 : Product
  To Workspace1 : ToWorkspace  VariableName=dampingTorque  SaveFormat=Timeseries  SampleTime=-1
  To Workspace4 : ToWorkspace  VariableName=passiveTorque  SaveFormat=Timeseries  SampleTime=-1
  Net External Torque : Outport
  wires:
  Velocity/1 -> Product3/1, Passive torque/2(Velocity)
  Global Damping/1 -> Product3/2  "Damping"
  Product3/1 -> Add/1, To Workspace1/1  "Damping torque"
  Position/1 -> Passive torque/1(Angle)
  Passive torque/1(Out1) -> Add/2, To Workspace4/1
  Add/1 -> Net External Torque/1

== system InteractiveArmModel_R2021a_v1/While Loop (Main Simulation Code)/Rigid Body Dynamics ==
  note: Output
  note: Input
  note: Angular convention:
      | arm angle is with respect to the left horizontal.
      | It's 0 degrees when aligned with the left horizontal.
      | Arm angle:
      | positive change: clockwise
      | Negative change: Counterclockwise
  Resultant torque : Inport
  Inertia : Constant  Value=0.007
  Product4 : Product
  Reciprocal : Product  Inputs=/  RndMeth=Zero  SaturateOnIntegerOverflow=on
  " Acceleration" : Outport
  wires:
  Product4/1 -> " Acceleration"/1  "Acceleration"
  Reciprocal/1 -> Product4/2
  Inertia/1 -> Reciprocal/1
  Resultant torque/1 -> Product4/1

== system InteractiveArmModel_R2021a_v1/While Loop (Main Simulation Code)/Stopping Logic ==
  Velocity (rad/s) : Inport
  Angle (radians) : Inport  Port=2
  Abs1 : Abs
  Abs2 : Abs
  GetTargetLocation : FunctionCaller  FunctionPrototype=y = Constants.targetLoc()  InputArgumentSpecifications=<Enter example>  OutputArgumentSpecifications=<Enter example>
  GetTargetLocation1 : FunctionCaller  FunctionPrototype=y = Constants.errorThresh()  InputArgumentSpecifications=<Enter example>  OutputArgumentSpecifications=<Enter example>
  GetVelocityThreshold : FunctionCaller  FunctionPrototype=y = Constants.velThresh()  InputArgumentSpecifications=<Enter example>  OutputArgumentSpecifications=<Enter example>
  Logical Operator : Logic  Operator=OR  AllPortsSameDT=off  OutDataTypeStr=boolean
  Relational Operator1 : RelationalOperator  Operator=>  OutDataTypeStr=boolean  RndMeth=Simplest
  Relational Operator2 : RelationalOperator  Operator=>  OutDataTypeStr=boolean  RndMeth=Simplest
  Subtract1 : Sum  Inputs=+-
  Out2 : Outport
  wires:
  Logical Operator/1 -> Out2/1  "StimCriteriaSatisfied"
  Relational Operator2/1 -> Logical Operator/2
  Abs2/1 -> Relational Operator1/1
  Abs1/1 -> Relational Operator2/1
  GetTargetLocation/1 -> Subtract1/1
  Subtract1/1 -> Abs1/1
  GetTargetLocation1/1 -> Relational Operator2/2
  GetVelocityThreshold/1 -> Relational Operator1/2
  Relational Operator1/1 -> Logical Operator/1
  Velocity (rad/s)/1 -> Abs2/1
  Angle (radians)/1 -> Subtract1/2

== system InteractiveArmModel_R2021a_v1/While Loop (Main Simulation Code)/Torque Gen. ==
  Torque(F&E) : Inport
  Constant : Constant  Value=-1
  Demux : Demux  Outputs=2
  Extensor Torque Generator Strength (Nm) : Constant  Value=2
  Flexor Torque Generator Strength (Nm) : Constant  Value=2
  Mux : Mux  Inputs=2
  Product : Product
  Product1 : Product
  Product2 : Product
  Torque (flex+Ext) : Outport
  wires:
  Product/1 -> Mux/2  "Extensor Torque"
  Extensor Torque Generator Strength (Nm)/1 -> Product/2
  Demux/1 -> Product1/1  "Flexor Torque (Nm)"
  Flexor Torque Generator Strength (Nm)/1 -> Product1/2
  Product1/1 -> Mux/1  "Flexor Torque"
  Torque(F&E)/1 -> Demux/1
  Mux/1 -> Torque (flex+Ext)/1
  Product2/1 -> Product/1  "Extensor Torque"
  Demux/2 -> Product2/1  "Extensor Torque (Nm)"
  Constant/1 -> Product2/2

== system InteractiveArmModel_R2021a_v1/Zero if Arm Not Active/If Action Subsystem1 ==
  In1 : Inport
  Action Port : ActionPort  ActionPortLabel=if(u1 == 0)
  Out1 : Outport
  wires:
  In1/1 -> Out1/1

== system InteractiveArmModel_R2021a_v1/Zero if Arm Not Active/If Action Subsystem10 ==
  In1 : Inport
  Action Port : ActionPort  ActionPortLabel=if(u1 == 0)
  Out1 : Outport
  wires:
  In1/1 -> Out1/1

== system InteractiveArmModel_R2021a_v1/Zero if Arm Not Active/If Action Subsystem11 ==
  " " : Inport
  Action Port : ActionPort  ActionPortLabel=else
  Out1 : Outport
  wires:
  " "/1 -> Out1/1

== system InteractiveArmModel_R2021a_v1/Zero if Arm Not Active/If Action Subsystem2 ==
  " " : Inport
  Action Port : ActionPort  ActionPortLabel=else
  Out1 : Outport
  wires:
  " "/1 -> Out1/1

== system InteractiveArmModel_R2021a_v1/Muscle_Mechanics_Functions/Contractile Element Excitation-Activation Relation/If Action Subsystem ==
  In1 : Inport
  Action Port : ActionPort  ActionPortLabel=if(u2>u1)
  Out1 : Outport
  wires:
  In1/1 -> Out1/1

== system InteractiveArmModel_R2021a_v1/Muscle_Mechanics_Functions/Contractile Element Excitation-Activation Relation/If Action Subsystem1 ==
  In1 : Inport
  Action Port : ActionPort  ActionPortLabel=elseif(u1>u2)
  Out1 : Outport
  wires:
  In1/1 -> Out1/1

== system InteractiveArmModel_R2021a_v1/Muscle_Mechanics_Functions/Contractile Element Excitation-Activation Relation/If Action Subsystem2 ==
  In1 : Inport
  Action Port : ActionPort  ActionPortLabel=else
  Out1 : Outport
  wires:
  In1/1 -> Out1/1

== system InteractiveArmModel_R2021a_v1/Muscle_Mechanics_Functions/Contractile Element Force-Length Relation/Force-length Relationship ==
  note: Output
  note: Inputs
  note: Constant
  In1 : Inport
  In2 : Inport  Port=2
  Constant1 : Constant
  Constant2 : Constant  Value=100
  Constant4 : Constant
  Display : Display
  Display1 : Display
  Divide : Product  Inputs=*/
  Function Caller : FunctionCaller  FunctionPrototype=y = Constants.L0F()  InputArgumentSpecifications=<Enter example>  OutputArgumentSpecifications=<Enter example>
  Function Caller1 : FunctionCaller  FunctionPrototype=y = Constants.L0E()  InputArgumentSpecifications=<Enter example>  OutputArgumentSpecifications=<Enter example>
  Function Caller3 : FunctionCaller  FunctionPrototype=y = Constants.WF()  InputArgumentSpecifications=<Enter example>  OutputArgumentSpecifications=<Enter example>
  Function Caller4 : FunctionCaller  FunctionPrototype=y = Constants.WE()  InputArgumentSpecifications=<Enter example>  OutputArgumentSpecifications=<Enter example>
  Math Function : Math  Operator=square  SaturateOnIntegerOverflow=on
  Product1 : Product  Inputs=3
  Scope1 : Scope
  Subtract : Sum  Inputs=+-
  Subtract1 : Sum  Inputs=+-
  Switch : Switch  Criteria=u2 > Threshold  Threshold=1
  Switch1 : Switch  Criteria=u2 > Threshold  Threshold=1
  To Workspace1 : ToWorkspace  VariableName=optLenCC_Ext  SaveFormat=Timeseries  SampleTime=-1
  To Workspace10 : ToWorkspace  VariableName=optLenCC_Flex  SaveFormat=Timeseries  SampleTime=-1
  FL : Outport
  W : Outport  Port=2
  L0 : Outport  Port=3
  wires:
  In1/1 -> Divide/1  "L_CE"
  Switch/1 -> Divide/2, L0/1  "L0"
  Divide/1 -> Subtract/1
  Constant1/1 -> Subtract/2
  Subtract/1 -> Math Function/1
  Math Function/1 -> Product1/1
  Constant2/1 -> Product1/2
  Switch1/1 -> Product1/3, W/1  "W"
  Product1/1 -> Subtract1/2
  Subtract1/1 -> FL/1, Scope1/1  "FL"
  Constant4/1 -> Subtract1/1
  Function Caller/1 -> To Workspace10/1, Display/1, Switch/1
  Function Caller1/1 -> To Workspace1/1, Display1/1, Switch/3
  In2/1 -> Switch1/2, Switch/2
  Function Caller4/1 -> Switch1/3
  Function Caller3/1 -> Switch1/1

== system InteractiveArmModel_R2021a_v1/Muscle_Mechanics_Functions/Contractile Element Force-Length Relation/If Action Subsystem ==
  In1 : Inport
  Action Port : ActionPort  ActionPortLabel=if(u1 > 0)
  Out1 : Outport
  wires:
  In1/1 -> Out1/1

== system InteractiveArmModel_R2021a_v1/Muscle_Mechanics_Functions/Contractile Element Force-Length Relation/If Action Subsystem1 ==
  In1 : Inport
  Action Port : ActionPort  ActionPortLabel=else
  Out1 : Outport
  wires:
  In1/1 -> Out1/1

== system InteractiveArmModel_R2021a_v1/Muscle_Mechanics_Functions/Contractile Element Force-Length Relation/If Action Subsystem10 ==
  In1 : Inport
  Action Port : ActionPort  ActionPortLabel=else
  Out1 : Outport
  wires:
  In1/1 -> Out1/1

== system InteractiveArmModel_R2021a_v1/Muscle_Mechanics_Functions/Contractile Element Force-Length Relation/If Action Subsystem2 ==
  In1 : Inport
  Action Port : ActionPort  ActionPortLabel=if(u1 == 1)
  Out1 : Outport
  wires:
  In1/1 -> Out1/1

== system InteractiveArmModel_R2021a_v1/Muscle_Mechanics_Functions/Contractile Element Force-Length Relation/If Action Subsystem3 ==
  In1 : Inport
  Action Port : ActionPort  ActionPortLabel=elseif(u2 == 1)
  Out1 : Outport
  wires:
  In1/1 -> Out1/1

== system InteractiveArmModel_R2021a_v1/Muscle_Mechanics_Functions/Contractile Element Force-Length Relation/If Action Subsystem4 ==
  In1 : Inport
  Action Port : ActionPort  ActionPortLabel=else
  Out1 : Outport
  wires:
  In1/1 -> Out1/1

== system InteractiveArmModel_R2021a_v1/Muscle_Mechanics_Functions/Contractile Element Force-Length Relation/If Action Subsystem5 ==
  In1 : Inport
  Action Port : ActionPort  ActionPortLabel=if(u1 > 0.00000001)
  Out1 : Outport
  wires:
  In1/1 -> Out1/1

== system InteractiveArmModel_R2021a_v1/Muscle_Mechanics_Functions/Contractile Element Force-Length Relation/If Action Subsystem6 ==
  In1 : Inport
  Action Port : ActionPort  ActionPortLabel=else
  Out1 : Outport
  wires:
  In1/1 -> Out1/1

== system InteractiveArmModel_R2021a_v1/Muscle_Mechanics_Functions/Contractile Element Force-Length Relation/If Action Subsystem7 ==
  In1 : Inport
  Action Port : ActionPort  ActionPortLabel=if(u1 > 0.00000001)
  Out1 : Outport
  wires:
  In1/1 -> Out1/1

== system InteractiveArmModel_R2021a_v1/Muscle_Mechanics_Functions/Contractile Element Force-Length Relation/If Action Subsystem8 ==
  In1 : Inport
  Action Port : ActionPort  ActionPortLabel=else
  Out1 : Outport
  wires:
  In1/1 -> Out1/1

== system InteractiveArmModel_R2021a_v1/Muscle_Mechanics_Functions/Contractile Element Force-Length Relation/If Action Subsystem9 ==
  In1 : Inport
  Action Port : ActionPort  ActionPortLabel=if(u1 == 0)
  Out1 : Outport
  wires:
  In1/1 -> Out1/1

== system InteractiveArmModel_R2021a_v1/Muscle_Mechanics_Functions/Contractile Element Force-Length Relation/L_calculation ==
  In1 : Inport
  Add : Sum
  Constant : Constant  Value=0.1
  Constant2 : Constant  Value=-1
  Constant3 : Constant  Value=10
  Constant4 : Constant
  Constant5 : Constant
  Constant6 : Constant  Value=100
  Divide : Product  Inputs=*/
  Product{1..4} (4 alike) : Product
  Scope1 : Scope  NumInputPorts=2
  Square Root : Sqrt  SaturateOnIntegerOverflow=on
  Subtract : Sum  Inputs=+-
  Subtract1 : Sum  Inputs=+-
  Out1 : Outport
  Out2 : Outport  Port=2
  wires:
  In1/1 -> Product4/1, Product3/1, Add/1  "PCoeff1"
  Constant2/1 -> Product3/2
  Constant/1 -> Product1/2  "rf"
  Add/1 -> Square Root/1
  Constant3/1 -> Product2/2
  Product3/1 -> Product2/1, Product1/1  "-pcoeff"
  Product1/1 -> Add/2
  Product2/1 -> Divide/2
  Square Root/1 -> Divide/1
  Divide/1 -> Subtract/2
  Constant4/1 -> Subtract/1
  Subtract/1 -> Subtract1/1  "L"
  Constant5/1 -> Subtract1/2
  Subtract1/1 -> Scope1/1, Out1/1  "L=L-1"
  Constant6/1 -> Product4/2
  Product4/1 -> Scope1/2, Out2/1  "C"

== system InteractiveArmModel_R2021a_v1/Muscle_Mechanics_Functions/Contractile Element Force-Length Relation/S1, S2, S3 calculation ==
  L : Inport
  C : Inport  Port=2
  normalised CC length : Inport  Port=3
  S1 : Subsystem
  S2 : Subsystem
  S3 : Subsystem
  S3 for condition 2 : Subsystem
  Out1 : Outport
  Out2 : Outport  Port=2
  Out3 : Outport  Port=3
  Out4 : Outport  Port=4
  wires:
  L/1 -> S1/1(In1), S2/1(In1), S3/1(In1)
  C/1 -> S2/2(In2), S1/2(In2), S3/2(In2)
  S1/1(Out1) -> S3/3(S1), S2/3(In3), Out1/1
  normalised CC length/1 -> S3/4(normalised CC length)
  S2/1(Out1) -> Out2/1
  S3/1(Out1) -> Out3/1
  S3/2(Out2) -> S3 for condition 2/1(In1)
  S3 for condition 2/1(Out1) -> Out4/1

== system InteractiveArmModel_R2021a_v1/Muscle_Mechanics_Functions/Contractile Element Force-Velocity Relation/CC is Isometric ==
  In1 : Inport
  Action Port : ActionPort  ActionPortLabel=elseif(u2 == 1)
  Out1 : Outport
  wires:
  In1/1 -> Out1/1

== system InteractiveArmModel_R2021a_v1/Muscle_Mechanics_Functions/Contractile Element Force-Velocity Relation/CC is Lengthening ==
  Vce : Inport
  Action Port : ActionPort  ActionPortLabel=else
  Out1 : Outport
  wires:
  Vce/1 -> Out1/1

== system InteractiveArmModel_R2021a_v1/Muscle_Mechanics_Functions/Contractile Element Force-Velocity Relation/CC is Shortening ==
  In1 : Inport
  Action Port : ActionPort  ActionPortLabel=if(u1 == 1)
  Out1 : Outport
  wires:
  In1/1 -> Out1/1

== system InteractiveArmModel_R2021a_v1/Muscle_Mechanics_Functions/Contractile Element Force-Velocity Relation/FP is non-zero ==
  In1 : Inport
  Action Port : ActionPort  ActionPortLabel=if(u1 > 0)
  Out1 : Outport
  wires:
  In1/1 -> Out1/1

== system InteractiveArmModel_R2021a_v1/Muscle_Mechanics_Functions/Contractile Element Force-Velocity Relation/FP<p ==
  note: Output
  note: Input
  note: Constants
  note: s
  FP : Inport
  P : Inport  Port=2
  E : Inport  Port=3
  a : Inport  Port=4
  b : Inport  Port=5
  Divide : Product  Inputs=*/
  Fiso+a : Sum
  Product1 : Product  Inputs=3
  Product2 : Product
  Subtract : Sum  Inputs=+-
  Subtract1 : Sum  Inputs=+-
  Subtract2 : Sum  Inputs=+-
  f_iso_ecc : Product
  f_iso_ecc2 : Product
  Vce : Outport
  wires:
  FP/1 -> Subtract/2, f_iso_ecc2/1, Subtract1/1, f_iso_ecc/1, Fiso+a/1
  E/1 -> f_iso_ecc2/2, f_iso_ecc/2
  f_iso_ecc2/1 -> Subtract/1
  Subtract/1 -> Product1/1
  b/1 -> Product1/3
  P/1 -> Subtract1/2, Subtract2/1
  Subtract1/1 -> Product1/2
  Product1/1 -> Divide/1
  a/1 -> Fiso+a/2
  Fiso+a/1 -> Product2/2
  f_iso_ecc/1 -> Subtract2/2
  Subtract2/1 -> Product2/1
  Product2/1 -> Divide/2
  Divide/1 -> Vce/1

== system InteractiveArmModel_R2021a_v1/Muscle_Mechanics_Functions/Contractile Element Force-Velocity Relation/FP>P ==
  note: Output
  note: Inputs
  FP : Inport
  P : Inport  Port=2
  a : Inport  Port=3
  b : Inport  Port=4
  Add : Sum
  Add1 : Sum
  Constant : Constant  Value=-1
  Divide : Product  Inputs=*/
  Product : Product
  Product1 : Product
  Subtract : Sum  Inputs=+-
  Vce : Outport
  wires:
  FP/1 -> Add/1
  a/1 -> Add1/2, Add/2
  Add/1 -> Product/1
  Product/1 -> Divide/1
  P/1 -> Add1/1
  Add1/1 -> Divide/2
  Divide/1 -> Subtract/1
  b/1 -> Subtract/2, Product/2
  Subtract/1 -> Product1/1
  Constant/1 -> Product1/2
  Product1/1 -> Vce/1

== system InteractiveArmModel_R2021a_v1/Muscle_Mechanics_Functions/Contractile Element Force-Velocity Relation/If Action Subsystem ==
  In1 : Inport
  Action Port : ActionPort  ActionPortLabel=if(u1 == 0)
  Out1 : Outport
  wires:
  In1/1 -> Out1/1

== system InteractiveArmModel_R2021a_v1/Muscle_Mechanics_Functions/Contractile Element Force-Velocity Relation/If Action Subsystem1 ==
  In1 : Inport
  Action Port : ActionPort  ActionPortLabel=else
  Out1 : Outport
  wires:
  In1/1 -> Out1/1

== system InteractiveArmModel_R2021a_v1/Muscle_Mechanics_Functions/Contractile Element Force-Velocity Relation/If Action Subsystem3 ==
  In1 : Inport
  Action Port : ActionPort  ActionPortLabel=else
  Out1 : Outport
  wires:
  In1/1 -> Out1/1

== system InteractiveArmModel_R2021a_v1/Muscle_Mechanics_Functions/Contractile Element Force-Velocity Relation/If Muscle Active ==
  In1 : Inport
  In2 : Inport  Port=2
  Action Port : ActionPort  ActionPortLabel=if(u1 > 0.001)
  Out1 : Outport
  Out2 : Outport  Port=2
  wires:
  In1/1 -> Out1/1
  In2/1 -> Out2/1

== system InteractiveArmModel_R2021a_v1/Muscle_Mechanics_Functions/Contractile Element Force-Velocity Relation/If Muscle NOT Active ==
  In1 : Inport
  In2 : Inport  Port=2
  Action Port : ActionPort  ActionPortLabel=else
  Out1 : Outport
  Out2 : Outport  Port=2
  wires:
  In1/1 -> Out1/1
  In2/1 -> Out2/1

== system InteractiveArmModel_R2021a_v1/Muscle_Mechanics_Functions/Contractile Element Force-Velocity Relation/dP//dt ==
  note: Output
  note: Input
  note: Constants
  Vsee : Inport
  alpha : Inport  Port=2
  P : Inport  Port=3
  beta : Inport  Port=4
  Po : Inport  Port=5
  Ls : Inport  Port=6
  Add : Sum
  Constant : Constant  Value=4
  Divide : Product  Inputs=*/
  Math Function : Math  Operator=square  SaturateOnIntegerOverflow=on
  Math Function1 : Math  Operator=square  SaturateOnIntegerOverflow=on
  Product : Product
  Product1 : Product  Inputs=4
  Product2 : Product
  Scope : Scope  NumInputPorts=2
  Square Root : Sqrt  SaturateOnIntegerOverflow=on
  dP/dt : Outport
  wires:
  P/1 -> Product1/3
  beta/1 -> Math Function/1
  Math Function1/1 -> Product/1
  Math Function/1 -> Product/2
  Constant/1 -> Product1/1
  Po/1 -> Product1/4, Math Function1/1
  alpha/1 -> Product1/2
  Product/1 -> Add/1
  Product1/1 -> Add/2
  Add/1 -> Square Root/1
  Square Root/1 -> Divide/1
  Ls/1 -> Divide/2
  Divide/1 -> Product2/2
  Vsee/1 -> Scope/2, Product2/1
  Product2/1 -> Scope/1, dP/dt/1  "dP/dt"

== system InteractiveArmModel_R2021a_v1/Muscle_Mechanics_Functions/Series-Elastic Element Stiffness Relation /If Action Subsystem ==
  In1 : Inport
  Action Port : ActionPort  ActionPortLabel=if(u1 == 0)
  Out1 : Outport
  wires:
  In1/1 -> Out1/1

== system InteractiveArmModel_R2021a_v1/Muscle_Mechanics_Functions/Series-Elastic Element Stiffness Relation /If Action Subsystem1 ==
  In1 : Inport
  Action Port : ActionPort  ActionPortLabel=else
  Out1 : Outport
  wires:
  In1/1 -> Out1/1

== system InteractiveArmModel_R2021a_v1/Trial Start//Stop//Increment Control/Flag for What Phase Trial is In/If Action Subsystem5 ==
  In1 : Inport
  Action Port : ActionPort  ActionPortLabel=if(u1 == 0)
  Out1 : Outport
  wires:
  In1/1 -> Out1/1
